simulink subsystem "EoM_3DoF"  (R2024b)
settings: Solver=VariableStepAuto  StartTime=0.0  StopTime=10.0  RelTol=1e-3
undefined symbols (not defined in the file or in its folder): com_error, inertia_error, mass_error, vehicle
settings Model: Creator=thatf  LastModifiedBy=alexa

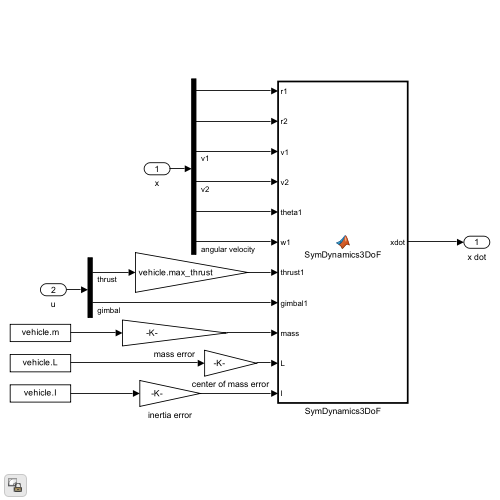
[thumbnail: Simulink's stored preview of the top-level diagram]
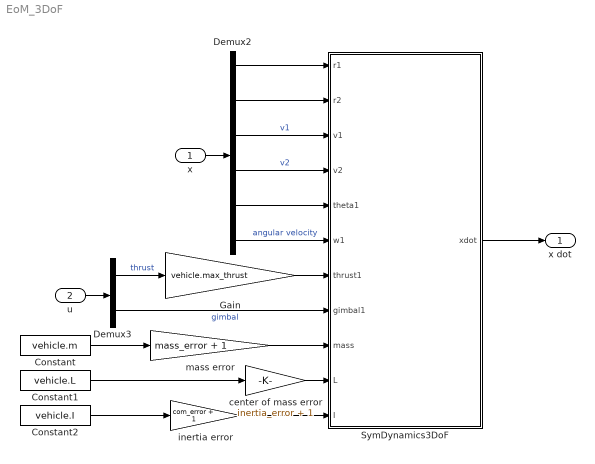
== system EoM_3DoF ==
  x : Inport
  u : Inport  Port=2
  Constant : Constant  Value=vehicle.m
  Constant1 : Constant  Value=vehicle.L
  Constant2 : Constant  Value=vehicle.I
  Demux2 : Demux  Outputs=6
  Demux3 : Demux  Outputs=2
  Gain : Gain  Gain=vehicle.max_thrust
  SymDynamics3DoF : MATLAB Function  TreatAsAtomicUnit=on
  center of mass error : Gain  Gain=inertia_error + 1
  inertia error : Gain  Gain=com_error + 1
  mass error : Gain  Gain=mass_error + 1
  x dot : Outport
  wires:
  u/1 -> Demux3/1
  x/1 -> Demux2/1
  Demux2/1 -> SymDynamics3DoF/1(r1)
  Demux2/2 -> SymDynamics3DoF/2(r2)
  Demux2/3 -> SymDynamics3DoF/3(v1)  "v1"
  Demux2/4 -> SymDynamics3DoF/4(v2)  "v2"
  Demux2/5 -> SymDynamics3DoF/5(theta1)
  Demux2/6 -> SymDynamics3DoF/6(w1)  "angular velocity"
  Demux3/2 -> SymDynamics3DoF/8(gimbal1)  "gimbal"
  Constant1/1 -> center of mass error/1
  Constant2/1 -> inertia error/1
  SymDynamics3DoF/1(xdot) -> x dot/1
  Gain/1 -> SymDynamics3DoF/7(thrust1)
  Demux3/1 -> Gain/1  "thrust"
  Constant/1 -> mass error/1
  center of mass error/1 -> SymDynamics3DoF/10(L)
  inertia error/1 -> SymDynamics3DoF/11(I)
  mass error/1 -> SymDynamics3DoF/9(mass)

== matlab function EoM_3DoF/SymDynamics3DoF ==
  data: r1 input; xdot output; r2 input; v1 input; v2 input; theta1 input; w1 input; thrust1 input; gimbal1 input; mass input; L input; I input
function xdot = SymDynamics3DoF(r1,r2,v1,v2,theta1,w1,thrust1,gimbal1,mass,L,I)
%#codegen

%    This function was generated by the Symbolic Math Toolbox version 24.2.
%    05-Nov-2024 14:06:10

% r1 = complex(r1);  % if required to enforce complex operations
% r2 = complex(r2);  % if required to enforce complex operations
% v1 = complex(v1);  % if required to enforce complex operations
% v2 = complex(v2);  % if required to enforce complex operations
% theta1 = complex(theta1);  % if required to enforce complex operations
% w1 = complex(w1);  % if required to enforce complex operations
% thrust1 = complex(thrust1);  % if required to enforce complex operations
% gimbal1 = complex(gimbal1);  % if required to enforce complex operations
% mass = complex(mass);  % if required to enforce complex operations
% L = complex(L);  % if required to enforce complex operations
% I = complex(I);  % if required to enforce complex operations
t2 = gimbal1+theta1;
t3 = 1.0./mass;
xdot = [v1;v2;t3.*thrust1.*cos(t2);t3.*thrust1.*sin(t2)-9.81e+2./1.0e+2;w1;-(L.*thrust1.*sin(gimbal1))./I];
end
